simulink model "untitled_R2015a"  (R2020b)
settings: Solver=VariableStepAuto  StartTime=0.0  StopTime=10.0  RelTol=1e-3
settings Model: Creator=tomonori  LastModifiedBy=tomonori
settings DebuggingCC: SFMachineParentedDataDiag=error

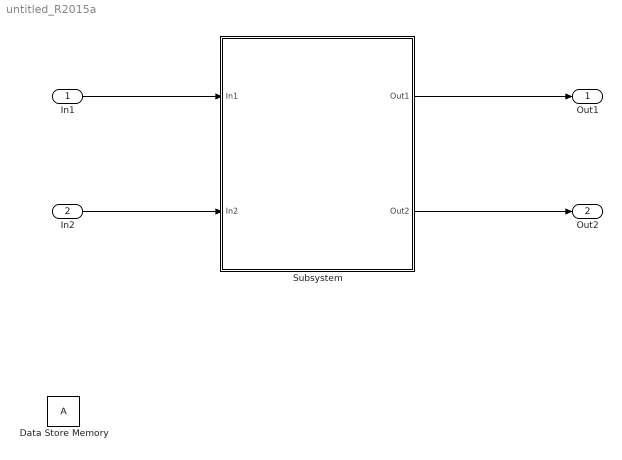
== system untitled_R2015a ==
  In1 : Inport
  In2 : Inport  Port=2
  Data Store Memory : DataStoreMemory  ReadBeforeWriteMsg=warning  WriteAfterWriteMsg=warning  WriteAfterReadMsg=warning  ShowAdditionalParam=off
  Subsystem : Subsystem
  Out1 : Outport
  Out2 : Outport  Port=2
  wires:
  In1/1 -> Subsystem/1(In1)
  Subsystem/1(Out1) -> Out1/1
  In2/1 -> Subsystem/2(In2)
  Subsystem/2(Out2) -> Out2/1

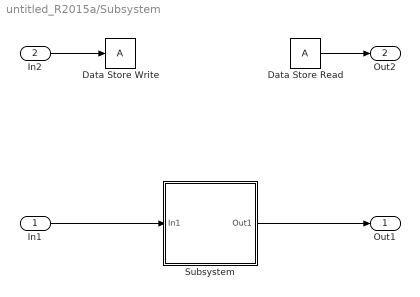
== system untitled_R2015a/Subsystem ==
  In1 : Inport
  In2 : Inport  Port=2
  Data Store Read : DataStoreRead
  Data Store Write : DataStoreWrite
  Subsystem : Subsystem  Variant=on  VariantControl=Choice
  Out1 : Outport
  Out2 : Outport  Port=2
  wires:
  In2/1 -> Data Store Write/1
  Data Store Read/1 -> Out2/1
  In1/1 -> Subsystem/1(In1)
  Subsystem/1(Out1) -> Out1/1

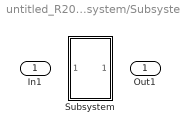
== system untitled_R2015a/Subsystem/Subsystem ==
  In1 : Inport
  Subsystem : Subsystem  TreatAsAtomicUnit=on  VariantControl=test_mode==1
  Out1 : Outport

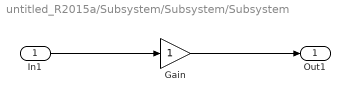
== system untitled_R2015a/Subsystem/Subsystem/Subsystem ==
  In1 : Inport
  Gain : Gain
  Out1 : Outport
  wires:
  Gain/1 -> Out1/1
  In1/1 -> Gain/1
